simulink model "PruebaLogicaIndices"  (R2022a)
settings: Solver=VariableStepAuto  StartTime=0.0  StopTime=inf  RelTol=1e-3
settings Model: Creator=user  LastModifiedBy=user

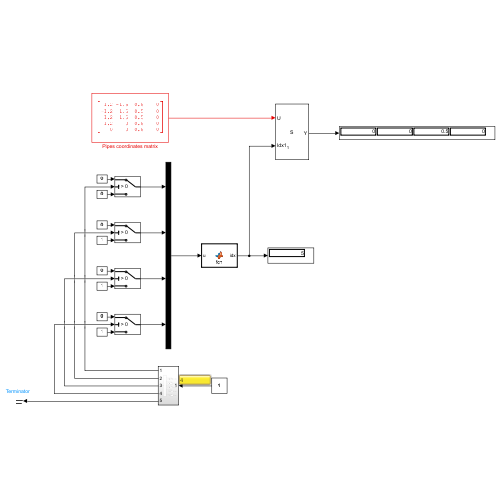
[thumbnail: Simulink's stored preview of the top-level diagram]
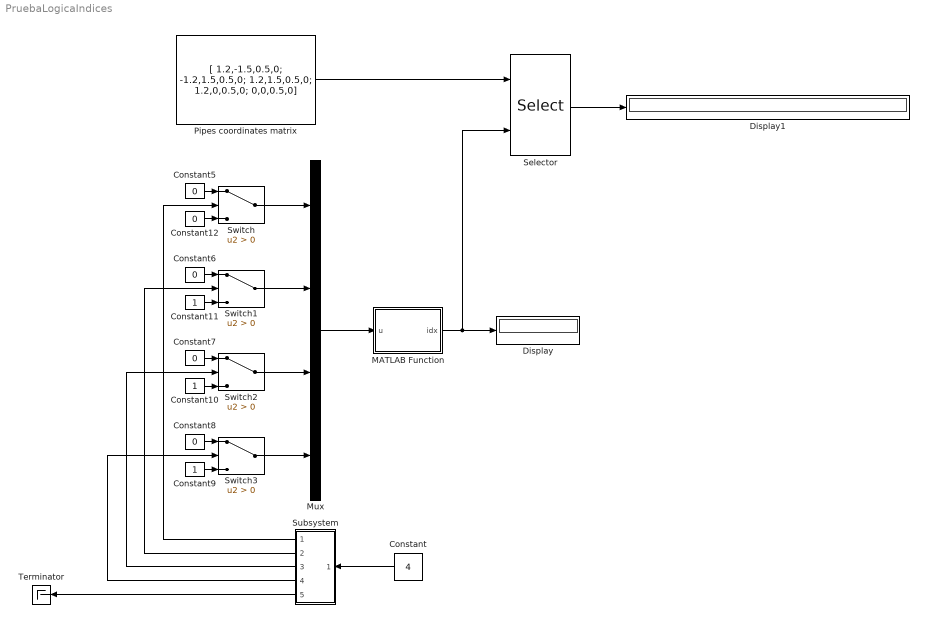
== system PruebaLogicaIndices ==
  Constant : Constant  Value=4
  Constant10 : Constant
  Constant11 : Constant
  Constant{5..8,12} (5 alike) : Constant  Value=0
  Constant9 : Constant
  Display : Display
  Display1 : Display
  MATLAB Function : MATLAB Function  TreatAsAtomicUnit=on
  Mux : Mux
  Pipes coordinates matrix : Constant  Value=[ 1.2,-1.5,0.5,0; -1.2,1.5,0.5,0; 1.2,1.5,0.5,0; 1.2,0,0.5,0; 0,0,0.5,0]  VectorParams1D=off
  Selector : Selector  NumberOfDimensions=2  InputPortWidth=3  IndexOptions=Starting index (port),Select all  Indices=[1 3],1  OutputSizes=1,1
  Subsystem : Subsystem
  Switch{,1..3} (4 alike) : Switch  Criteria=u2 > Threshold  SaturateOnIntegerOverflow=off  InputSameDT=off
  Terminator : Terminator
  wires:
  Constant5/1 -> Switch/1
  Constant6/1 -> Switch1/1
  Constant7/1 -> Switch2/1
  Constant8/1 -> Switch3/1
  Constant9/1 -> Switch3/3
  Constant10/1 -> Switch2/3
  Constant11/1 -> Switch1/3
  Constant12/1 -> Switch/3
  Mux/1 -> MATLAB Function/1(u)
  Pipes coordinates matrix/1 -> Selector/1
  MATLAB Function/1(idx) -> Display/1, Selector/2
  Switch/1 -> Mux/1
  Switch1/1 -> Mux/2
  Switch2/1 -> Mux/3
  Switch3/1 -> Mux/4
  Selector/1 -> Display1/1
  Subsystem/1(Out1) -> Switch/2
  Subsystem/2(Out2) -> Switch1/2
  Subsystem/3(Out3) -> Switch2/2
  Subsystem/4(Out4) -> Switch3/2
  Subsystem/5(Out5) -> Terminator/1
  Constant/1 -> Subsystem/1(In1)

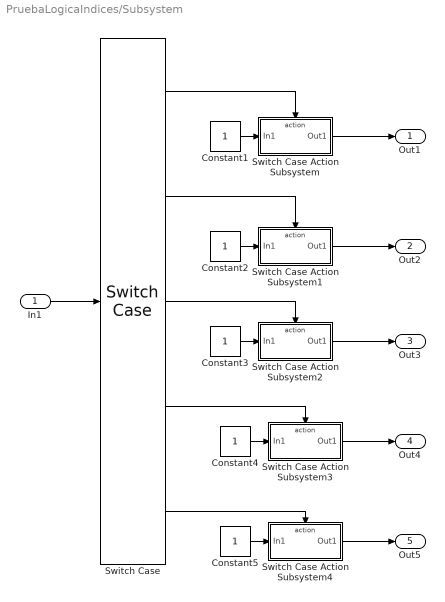
== system PruebaLogicaIndices/Subsystem ==
  In1 : Inport
  Constant{1..5} (5 alike) : Constant
  Switch Case : SwitchCase  CaseConditions={1,2,3,4}
  Switch Case Action Subsystem : Subsystem  TreatAsAtomicUnit=on
  Switch Case Action Subsystem1 : Subsystem  TreatAsAtomicUnit=on
  Switch Case Action Subsystem2 : Subsystem  TreatAsAtomicUnit=on
  Switch Case Action Subsystem3 : Subsystem  TreatAsAtomicUnit=on
  Switch Case Action Subsystem4 : Subsystem  TreatAsAtomicUnit=on
  Out1 : Outport
  Out2 : Outport  Port=2
  Out3 : Outport  Port=3
  Out4 : Outport  Port=4
  Out5 : Outport  Port=5
  wires:
  Switch Case/1 -> Switch Case Action Subsystem/Action
  Switch Case/3 -> Switch Case Action Subsystem2/Action
  Constant4/1 -> Switch Case Action Subsystem3/1(In1)
  Constant3/1 -> Switch Case Action Subsystem2/1(In1)
  Constant2/1 -> Switch Case Action Subsystem1/1(In1)
  Switch Case/4 -> Switch Case Action Subsystem3/Action
  Switch Case Action Subsystem2/1(Out1) -> Out3/1
  Switch Case/2 -> Switch Case Action Subsystem1/Action
  Constant1/1 -> Switch Case Action Subsystem/1(In1)
  Switch Case Action Subsystem1/1(Out1) -> Out2/1
  Switch Case Action Subsystem/1(Out1) -> Out1/1
  In1/1 -> Switch Case/1
  Switch Case Action Subsystem3/1(Out1) -> Out4/1
  Switch Case Action Subsystem4/1(Out1) -> Out5/1
  Constant5/1 -> Switch Case Action Subsystem4/1(In1)
  Switch Case/5 -> Switch Case Action Subsystem4/Action

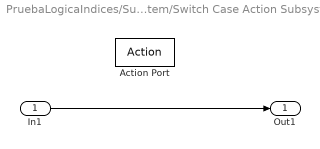
== system PruebaLogicaIndices/Subsystem/Switch Case Action Subsystem ==
  In1 : Inport
  Action Port : ActionPort  ActionPortLabel=case [ 1 ]:
  Out1 : Outport
  wires:
  In1/1 -> Out1/1

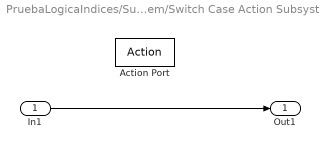
== system PruebaLogicaIndices/Subsystem/Switch Case Action Subsystem1 ==
  In1 : Inport
  Action Port : ActionPort  ActionPortLabel=case [ 2 ]:
  Out1 : Outport
  wires:
  In1/1 -> Out1/1

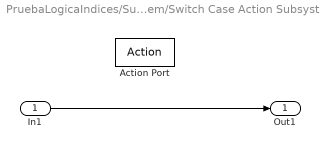
== system PruebaLogicaIndices/Subsystem/Switch Case Action Subsystem2 ==
  In1 : Inport
  Action Port : ActionPort  ActionPortLabel=case [ 3 ]:
  Out1 : Outport
  wires:
  In1/1 -> Out1/1

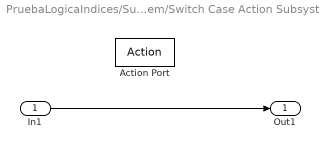
== system PruebaLogicaIndices/Subsystem/Switch Case Action Subsystem3 ==
  In1 : Inport
  Action Port : ActionPort  ActionPortLabel=case [ 4 ]:
  Out1 : Outport
  wires:
  In1/1 -> Out1/1

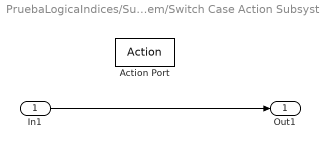
== system PruebaLogicaIndices/Subsystem/Switch Case Action Subsystem4 ==
  In1 : Inport
  Action Port : ActionPort  ActionPortLabel=default:
  Out1 : Outport
  wires:
  In1/1 -> Out1/1

== matlab function PruebaLogicaIndices/MATLAB Function ==
  data: u input; idx output
function idx = fcn(u)

indexes = find(u,1,'first');

if isempty(indexes)
    idx = 5;
else
    idx = indexes(1);
end
